simulink model "Zdomain"  (R2023b)
settings: Solver=VariableStepAuto  StartTime=0.0  StopTime=100  RelTol=1e-3
undefined symbols (not defined in the file): DiscIntNeverNeededParam
libraries: simulink x1, cstblocks x1
settings Model: Creator=Administrator  LastModifiedBy=Administrator

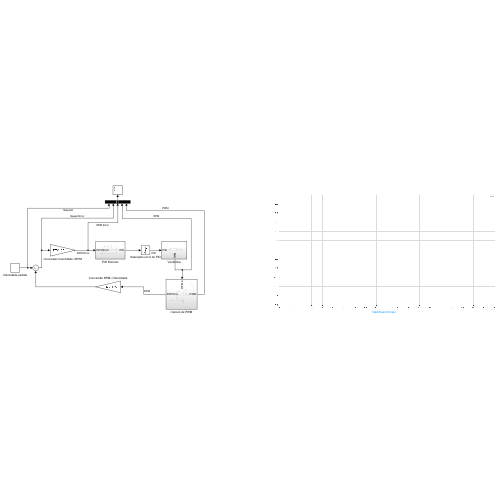
[thumbnail: Simulink's stored preview of the top-level diagram]
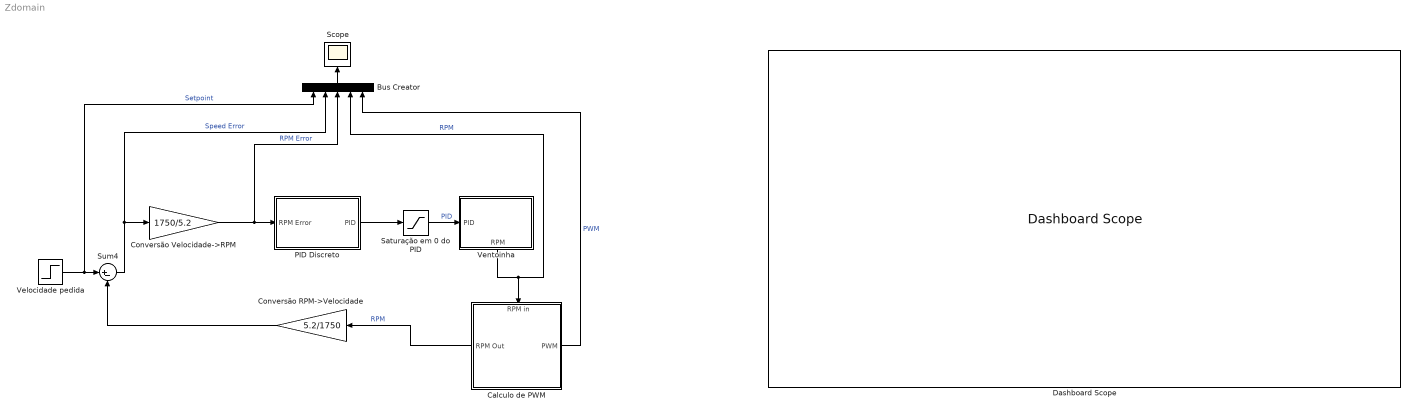
== system Zdomain ==
  Bus Creator : BusCreator  Inputs=5
  Calculo de PWM : Subsystem
      settings: PortSchema="{\"entries\":[{\"content\":{\"sides\":[{\"content\":{\"connectorIds\":[\"Out2\"]},\"type\":\"ConnectorPlacement.EquallySpacedRectSide\",\"uuid\":\"a240e75c-ea08-4aa3-822f-b73cad036c4a\"},{\"content\":{\"connectorIds\":[\"Out1\"],\"side\":\"RIGHT\"},\"type\":\"ConnectorPlacement.EquallySpacedRectSide\",\"uuid\":\"da6ac24d-a89c-4014-9688-266e0e62c615\"},{\"content\":{\"connectorIds\":[\"In1\"],\"side\":\"TOP\"},\"type\":\"ConnectorPlacement.EquallySpacedRectSide\",\"uuid\":\"4ed089fe-ce6e-49a1-a8f0-9d77dc88e234\"}]},\"type\":\"ConnectorPlacement.EquallySpacedConnector\",\"uuid\":\"baa3b966-1298-4d18-b102-d98e79f1aa87\"}],\"packageUris\":[\"http://schema.mathworks.com/mf0/Connector/R2020b\"],\"version\":\"1.0\"}"
  Conversão RPM->Velocidade : Gain  Gain=5.2/1750
  Conversão Velocidade->RPM : Gain  Gain=1750/5.2
  Dashboard Scope : DashboardScope
  PID Discreto : Subsystem
  Saturação em 0 do PID : Saturate  UpperLimit=10000  LowerLimit=0
  Scope : Scope
  Sum4 : Sum  Inputs=|+-
  Velocidade pedida : Step  After=7  SampleTime=0
  Ventoinha : Subsystem
      settings: PortSchema="{\"entries\":[{\"content\":{\"sides\":[{\"content\":{\"connectorIds\":[\"In1\"]},\"type\":\"ConnectorPlacement.EquallySpacedRectSide\",\"uuid\":\"b947db97-fa09-4e3b-b416-4cd776b95088\"},{\"content\":{\"side\":\"RIGHT\"},\"type\":\"ConnectorPlacement.EquallySpacedRectSide\",\"uuid\":\"db74d998-fecc-49fa-b45f-57676d45925c\"},{\"content\":{\"side\":\"TOP\"},\"type\":\"ConnectorPlacement.EquallySpacedRectSide\",\"uuid\":\"dcd3bfb3-f90e-48a9-9950-5faafc442ba9\"},{\"content\":{\"connectorIds\":[\"Out1\"],\"side\":\"BOTTOM\"},\"type\":\"ConnectorPlacement.EquallySpacedRectSide\",\"uuid\":\"0695d77e-9243-4108-8141-ab881e35d38e\"}]},\"type\":\"ConnectorPlacement.EquallySpacedConnector\",\"uuid\":\"2df329e1-957b-4b7e-9af2-b4ef73900dda\"}],\"packageUris\":[\"http://schema.mathworks.com/mf0/Connector/R2020b\"],\"version\":\"1.0\"}"
  wires:
  Sum4/1 -> Bus Creator/2, Conversão Velocidade->RPM/1  "Speed Error"
  Velocidade pedida/1 -> Bus Creator/1, Sum4/1  "Setpoint"
  Conversão Velocidade->RPM/1 -> PID Discreto/1(RPM Error), Bus Creator/3  "RPM Error"
  Bus Creator/1 -> Scope/1
  Conversão RPM->Velocidade/1 -> Sum4/2
  Calculo de PWM/2(PWM) -> Bus Creator/5  "PWM"
  Calculo de PWM/1(RPM Out) -> Conversão RPM->Velocidade/1  "RPM"
  Ventoinha/1(RPM) -> Bus Creator/4, Calculo de PWM/1(RPM in)  "RPM"
  Saturação em 0 do PID/1 -> Ventoinha/1(PID)  "PID"
  PID Discreto/1(PID) -> Saturação em 0 do PID/1

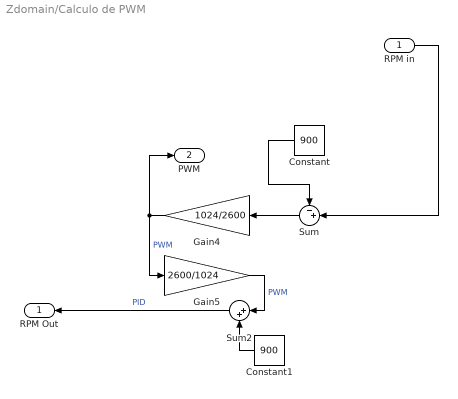
== system Zdomain/Calculo de PWM ==
  RPM in : Inport
  Constant : Constant  Value=900
  Constant1 : Constant  Value=900
  Gain4 : Gain  Gain=1024/2600
  Gain5 : Gain  Gain=2600/1024
  Sum : Sum  Inputs=-+|
  Sum2 : Sum  Inputs=|++
  RPM Out : Outport
  PWM : Outport  Port=2
  wires:
  Gain4/1 -> Gain5/1, PWM/1  "PWM"
  Sum/1 -> Gain4/1
  RPM in/1 -> Sum/2
  Constant1/1 -> Sum2/2
  Constant/1 -> Sum/1
  Sum2/1 -> RPM Out/1  "PID"
  Gain5/1 -> Sum2/1  "PWM"

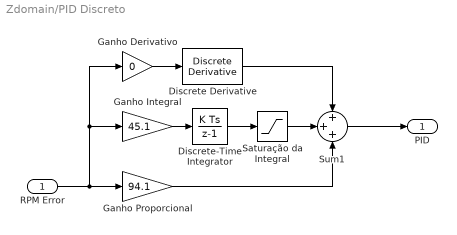
== system Zdomain/PID Discreto ==
  RPM Error : Inport
  Discrete Derivative : simulink/Discrete/Discrete Derivative  gainval=1.0  ICPrevScaledInput=0.0  OutMin=[]  OutMax=[]  OutDataType=fixdt(1, 16)  OutScaling=2^-10  DoSatur=off
  Discrete-Time Integrator : DiscreteIntegrator  SampleTime=-1  ICPrevOutput=DiscIntNeverNeededParam  ICPrevScaledInput=DiscIntNeverNeededParam
  Ganho Derivativo : Gain  Gain=0
  Ganho Integral : Gain  Gain=45.1
  Ganho Proporcional : Gain  Gain=94.1
  Saturação da Integral : Saturate  UpperLimit=10000  LowerLimit=0
  Sum1 : Sum  Inputs=+++
  PID : Outport
  wires:
  Sum1/1 -> PID/1
  Discrete Derivative/1 -> Sum1/1
  Saturação da Integral/1 -> Sum1/2
  RPM Error/1 -> Ganho Proporcional/1, Ganho Derivativo/1, Ganho Integral/1
  Ganho Derivativo/1 -> Discrete Derivative/1
  Ganho Proporcional/1 -> Sum1/3
  Ganho Integral/1 -> Discrete-Time Integrator/1
  Discrete-Time Integrator/1 -> Saturação da Integral/1

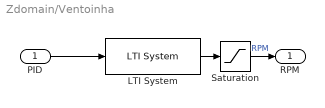
== system Zdomain/Ventoinha ==
  PID : Inport
  LTI System : cstblocks/LTI System  sys=sysZ  IC=[]  PadeOrder=0
  Saturation : Saturate  UpperLimit=3600  LowerLimit=900
  RPM : Outport
  wires:
  LTI System/1 -> Saturation/1
  PID/1 -> LTI System/1
  Saturation/1 -> RPM/1  "RPM"
